simulink model "p1_1"  (R2019b)
settings: Solver=VariableStepAuto  StartTime=0.0  StopTime=80.0  RelTol=1e-3
settings Model: Creator=ushio  LastModifiedBy=ushio

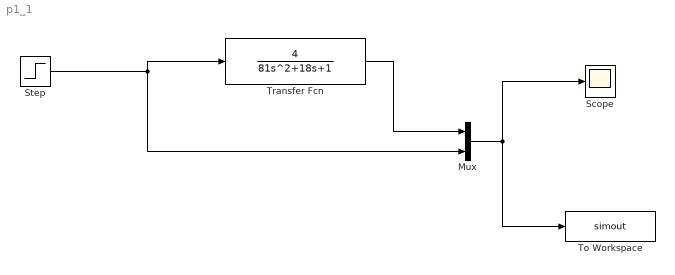
== system p1_1 ==
  Mux : Mux  Inputs=2
  Scope : Scope
  Step : Step  Time=0  SampleTime=0
  To Workspace : ToWorkspace  VariableName=simout  SaveFormat=Timeseries  SampleTime=-1
  Transfer Fcn : TransferFcn  Numerator=4  Denominator=[81 18 1]
  wires:
  Step/1 -> Transfer Fcn/1, Mux/2
  Transfer Fcn/1 -> Mux/1
  Mux/1 -> To Workspace/1, Scope/1
